simulink model "ASM_Traffic_V2X_Complete_Model_2"  (R2019a)
settings: Solver=ode1  StartTime=SIM.tstart.v  StopTime=Inf  FixedStep=SIM.StepSize.v  RelTol=1e-3
PostLoadFcn:
  | if any(exist('dsrtsu_mdlpostloadfcn', 'file') ~= 0), dsrtsu_mdlpostloadfcn('Execute', bdroot); end
  | try, asm_mdl_postloadfcn(bdroot, 'UpdateModel', 2200); catch, disp(lasterr); end,
undefined symbols (not defined in the file): _SensorPnts_1, _SensorPnts_13, _SensorPnts_17, _SensorPnts_21, _SensorPnts_25, _SensorPnts_29, _SensorPnts_33, _SensorPnts_37, _SensorPnts_41, _SensorPnts_45, _SensorPnts_49, _SensorPnts_5, _SensorPnts_53, _SensorPnts_57, _SensorPnts_9, _to_, CPT, G5A, ITS, MDL, rad, s_to_rpm, SIM
libraries: simulink x169, ASM_VehicleDynamics_lib x126, ASM_Traffic_lib x83, ASM_Utils_lib x49, mdbs x45, ASM_Environment_lib x17, dspindex x12, dsaV2xLibraryAux x10, dsmpblib x6, dsaV2xAsn1Library x4, dsaV2xLibrary x4, ASM_BrakeHydraulics_lib x4
(part 9 of 36)

== system ASM_Traffic_V2X_Complete_Model_2/MDLUserInterface/MotionDeskInterface/ASM_VehicleLights ==
  Environment : Inport
  VehDyn : Inport  Port=2
  Bus Selector : BusSelector  OutputSignals=Maneuver.UserSignals_Customized.ASM_Vehicle_TurnLights[]
  Bus Selector1 : BusSelector  OutputSignals=SW_ManualControl_Lights[1Maneuver|2Manual],SW_BrakeLight[0Off|1On],SW_TurnLights[0Off|1Left|2Right|3Both]
  Bus Selector3 : BusSelector  OutputSignals=Brake.BrakeDisc.Pressure.p_FL_Brake[bar],Brake.BrakeDisc.Pressure.p_FR_Brake[bar],Brake.BrakeDisc.Pressure.p_RL_Brake[bar],Brake.BrakeDisc.Pressure.p_RR_Brake[bar]
  Cmp_BrakePres : simulink/Logic and Bit Operations/Compare To Constant  relop=>  const=3  OutDataTypeStr=boolean
  Compare_Hazard : simulink/Logic and Bit Operations/Compare To Constant  relop===  const=3  OutDataTypeStr=boolean
  Compare_Turnlight_L : simulink/Logic and Bit Operations/Compare To Constant  relop===  const=1.0  OutDataTypeStr=boolean
  Compare_Turnlight_R : simulink/Logic and Bit Operations/Compare To Constant  relop===  const=2  OutDataTypeStr=boolean
  Data Type Conversion1 : DataTypeConversion  OutDataTypeStr=boolean
  Data Type Conversion2 : DataTypeConversion  OutDataTypeStr=uint32
  Data Type Conversion3 : DataTypeConversion  OutDataTypeStr=uint32
  Data Type Conversion4 : DataTypeConversion  OutDataTypeStr=uint32
  Gain : Gain  Gain=1/4
  Logical Operator : Logic  Operator=OR  AllPortsSameDT=off  OutDataTypeStr=boolean
  Logical Operator1 : Logic  Operator=OR  AllPortsSameDT=off  OutDataTypeStr=boolean
  Multiport Switch : MultiPortSwitch  Inputs=2
  Multiport Switch4 : MultiPortSwitch  Inputs=2
  Mux : Mux  Inputs=3
  Mux1 : Mux
  Sum of Elements : Sum  Inputs=+
  ASM_Vehicle_Lights[] : Outport
  wires:
  Mux/1 -> ASM_Vehicle_Lights[]/1
  Environment/1 -> Bus Selector/1
  Bus Selector/1 -> Data Type Conversion4/1  "<ASM_Vehicle_TurnLights[]>"
  Bus Selector1/1 -> Data Type Conversion3/1  "<SW_ManualControl_Lights[1Maneuver|2Manual]>"
  Bus Selector1/2 -> Data Type Conversion1/1  "<SW_BrakeLight[0Off|1On]>"
  Multiport Switch/1 -> Mux/1
  Compare_Turnlight_L/1 -> Logical Operator/1
  Compare_Turnlight_R/1 -> Logical Operator1/1
  Compare_Hazard/1 -> Logical Operator1/2, Logical Operator/2
  Logical Operator/1 -> Mux/2
  Logical Operator1/1 -> Mux/3
  Multiport Switch4/1 -> Compare_Turnlight_L/1, Compare_Turnlight_R/1, Compare_Hazard/1
  Bus Selector1/3 -> Data Type Conversion2/1  "<SW_TurnLights[0Off|1Left|2Right|3Both]>"
  [TAG_SW_ASMVehicleLights_Signals] -> Bus Selector1/1
  Data Type Conversion3/1 -> Multiport Switch/1, Multiport Switch4/1
  Data Type Conversion1/1 -> Multiport Switch/3
  Data Type Conversion2/1 -> Multiport Switch4/3
  Data Type Conversion4/1 -> Multiport Switch4/2
  VehDyn/1 -> Bus Selector3/1
  Cmp_BrakePres/1 -> Multiport Switch/2
  Bus Selector3/2 -> Mux1/2  "<p_FR_Brake[bar]>"
  Bus Selector3/4 -> Mux1/4  "<p_RR_Brake[bar]>"
  Bus Selector3/1 -> Mux1/1  "<p_FL_Brake[bar]>"
  Bus Selector3/3 -> Mux1/3  "<p_RL_Brake[bar]>"
  Sum of Elements/1 -> Gain/1
  Mux1/1 -> Sum of Elements/1
  Gain/1 -> Cmp_BrakePres/1

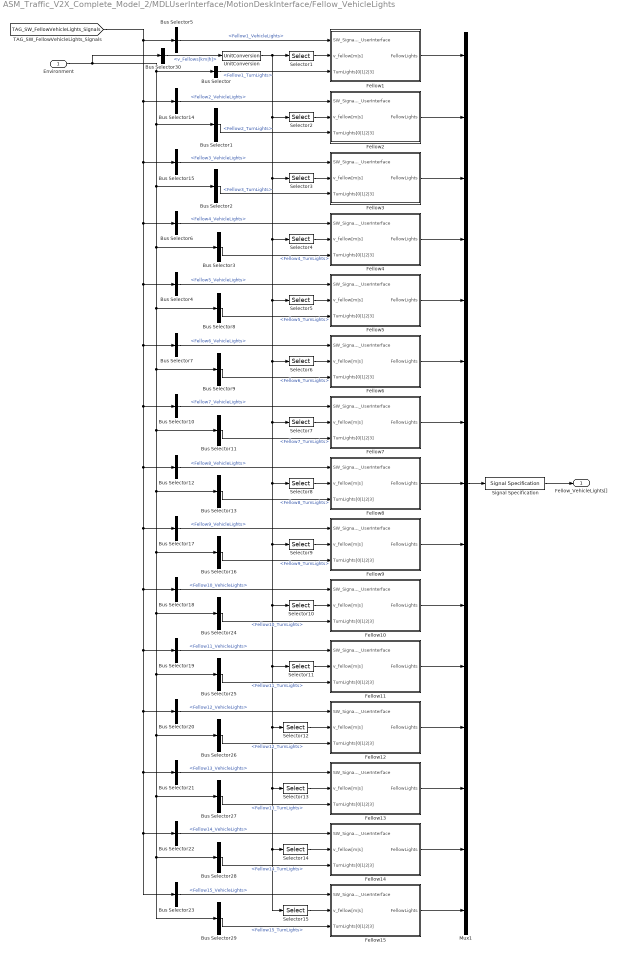
== system ASM_Traffic_V2X_Complete_Model_2/MDLUserInterface/MotionDeskInterface/Fellow_VehicleLights ==
  Environment : Inport
  Bus Selector : BusSelector  OutputSignals=Traffic.FellowMovement.UserSignals_Customized.Fellow1_TurnLights
  Bus Selector1 : BusSelector  OutputSignals=Traffic.FellowMovement.UserSignals_Customized.Fellow2_TurnLights
  Bus Selector10 : BusSelector  OutputSignals=Fellow7_VehicleLights
  Bus Selector11 : BusSelector  OutputSignals=Traffic.FellowMovement.UserSignals_Customized.Fellow7_TurnLights
  Bus Selector12 : BusSelector  OutputSignals=Fellow8_VehicleLights
  Bus Selector13 : BusSelector  OutputSignals=Traffic.FellowMovement.UserSignals_Customized.Fellow8_TurnLights
  Bus Selector14 : BusSelector  OutputSignals=Fellow2_VehicleLights
  Bus Selector15 : BusSelector  OutputSignals=Fellow3_VehicleLights
  Bus Selector16 : BusSelector  OutputSignals=Traffic.FellowMovement.UserSignals_Customized.Fellow9_TurnLights
  Bus Selector17 : BusSelector  OutputSignals=Fellow9_VehicleLights
  Bus Selector18 : BusSelector  OutputSignals=Fellow10_VehicleLights
  Bus Selector19 : BusSelector  OutputSignals=Fellow11_VehicleLights
  Bus Selector2 : BusSelector  OutputSignals=Traffic.FellowMovement.UserSignals_Customized.Fellow3_TurnLights
  Bus Selector20 : BusSelector  OutputSignals=Fellow12_VehicleLights
  Bus Selector21 : BusSelector  OutputSignals=Fellow13_VehicleLights
  Bus Selector22 : BusSelector  OutputSignals=Fellow14_VehicleLights
  Bus Selector23 : BusSelector  OutputSignals=Fellow15_VehicleLights
  Bus Selector24 : BusSelector  OutputSignals=Traffic.FellowMovement.UserSignals_Customized.Fellow10_TurnLights
  Bus Selector25 : BusSelector  OutputSignals=Traffic.FellowMovement.UserSignals_Customized.Fellow11_TurnLights
  Bus Selector26 : BusSelector  OutputSignals=Traffic.FellowMovement.UserSignals_Customized.Fellow12_TurnLights
  Bus Selector27 : BusSelector  OutputSignals=Traffic.FellowMovement.UserSignals_Customized.Fellow13_TurnLights
  Bus Selector28 : BusSelector  OutputSignals=Traffic.FellowMovement.UserSignals_Customized.Fellow14_TurnLights
  Bus Selector29 : BusSelector  OutputSignals=Traffic.FellowMovement.UserSignals_Customized.Fellow15_TurnLights
  Bus Selector3 : BusSelector  OutputSignals=Traffic.FellowMovement.UserSignals_Customized.Fellow4_TurnLights
  Bus Selector30 : BusSelector  OutputSignals=Traffic.FellowMovement.FellowMovement.v_Fellows[km|h]
  Bus Selector4 : BusSelector  OutputSignals=Fellow5_VehicleLights
  Bus Selector5 : BusSelector  OutputSignals=Fellow1_VehicleLights
  Bus Selector6 : BusSelector  OutputSignals=Fellow4_VehicleLights
  Bus Selector7 : BusSelector  OutputSignals=Fellow6_VehicleLights
  Bus Selector8 : BusSelector  OutputSignals=Traffic.FellowMovement.UserSignals_Customized.Fellow5_TurnLights
  Bus Selector9 : BusSelector  OutputSignals=Traffic.FellowMovement.UserSignals_Customized.Fellow6_TurnLights
  Fellow1 : Subsystem
  Fellow10 : Subsystem
  Fellow11 : Subsystem
  Fellow12 : Subsystem
  Fellow13 : Subsystem
  Fellow14 : Subsystem
  Fellow15 : Subsystem
  Fellow2 : Subsystem
  Fellow3 : Subsystem
  Fellow4 : Subsystem
  Fellow5 : Subsystem
  Fellow6 : Subsystem
  Fellow7 : Subsystem
  Fellow8 : Subsystem
  Fellow9 : Subsystem
  Mux1 : Mux  Inputs=15
  Selector1 : Selector  InputPortWidth=MDL.Traffic.MaxNumFellows.v  IndexOptions=Index vector (dialog)  Indices=1  OutputSizes=1
  Selector10 : Selector  InputPortWidth=MDL.Traffic.MaxNumFellows.v  IndexOptions=Index vector (dialog)  Indices=10  OutputSizes=1
  Selector11 : Selector  InputPortWidth=MDL.Traffic.MaxNumFellows.v  IndexOptions=Index vector (dialog)  Indices=11  OutputSizes=1
  Selector12 : Selector  InputPortWidth=MDL.Traffic.MaxNumFellows.v  IndexOptions=Index vector (dialog)  Indices=12  OutputSizes=1
  Selector13 : Selector  InputPortWidth=MDL.Traffic.MaxNumFellows.v  IndexOptions=Index vector (dialog)  Indices=13  OutputSizes=1
  Selector14 : Selector  InputPortWidth=MDL.Traffic.MaxNumFellows.v  IndexOptions=Index vector (dialog)  Indices=14  OutputSizes=1
  Selector15 : Selector  InputPortWidth=MDL.Traffic.MaxNumFellows.v  IndexOptions=Index vector (dialog)  Indices=15  OutputSizes=1
  Selector2 : Selector  InputPortWidth=MDL.Traffic.MaxNumFellows.v  IndexOptions=Index vector (dialog)  Indices=2  OutputSizes=1
  Selector3 : Selector  InputPortWidth=MDL.Traffic.MaxNumFellows.v  IndexOptions=Index vector (dialog)  Indices=3  OutputSizes=1
  Selector4 : Selector  InputPortWidth=MDL.Traffic.MaxNumFellows.v  IndexOptions=Index vector (dialog)  Indices=4  OutputSizes=1
  Selector5 : Selector  InputPortWidth=MDL.Traffic.MaxNumFellows.v  IndexOptions=Index vector (dialog)  Indices=5  OutputSizes=1
  Selector6 : Selector  InputPortWidth=MDL.Traffic.MaxNumFellows.v  IndexOptions=Index vector (dialog)  Indices=6  OutputSizes=1
  Selector7 : Selector  InputPortWidth=MDL.Traffic.MaxNumFellows.v  IndexOptions=Index vector (dialog)  Indices=7  OutputSizes=1
  Selector8 : Selector  InputPortWidth=MDL.Traffic.MaxNumFellows.v  IndexOptions=Index vector (dialog)  Indices=8  OutputSizes=1
  Selector9 : Selector  InputPortWidth=MDL.Traffic.MaxNumFellows.v  IndexOptions=Index vector (dialog)  Indices=9  OutputSizes=1
  Signal Specification : SignalSpecification  SampleTime=SIM.StepSize.v
  UnitConversion : ASM_Utils_lib/UnitConversion/UnitConversion  Selection=km/h_to_m/s
  Fellow_VehicleLights[] : Outport
  wires:
  UnitConversion/1 -> Selector1/1, Selector2/1, Selector3/1, Selector4/1, Selector5/1, Selector6/1, Selector7/1, Selector8/1, Selector9/1, Selector10/1, Selector11/1, Selector12/1, Selector13/1, Selector14/1, Selector15/1
  Bus Selector29/1 -> Fellow15/3(TurnLights[0|1|2|3])  "<Fellow15_TurnLights>"
  Bus Selector28/1 -> Fellow14/3(TurnLights[0|1|2|3])  "<Fellow14_TurnLights>"
  Bus Selector22/1 -> Fellow14/1(SW_Signals_UserInterface)  "<Fellow14_VehicleLights>"
  Bus Selector27/1 -> Fellow13/3(TurnLights[0|1|2|3])  "<Fellow13_TurnLights>"
  Bus Selector21/1 -> Fellow13/1(SW_Signals_UserInterface)  "<Fellow13_VehicleLights>"
  Bus Selector26/1 -> Fellow12/3(TurnLights[0|1|2|3])  "<Fellow12_TurnLights>"
  Bus Selector25/1 -> Fellow11/3(TurnLights[0|1|2|3])  "<Fellow11_TurnLights>"
  Bus Selector24/1 -> Fellow10/3(TurnLights[0|1|2|3])  "<Fellow10_TurnLights>"
  Bus Selector16/1 -> Fellow9/3(TurnLights[0|1|2|3])  "<Fellow9_TurnLights>"
  Bus Selector13/1 -> Fellow8/3(TurnLights[0|1|2|3])  "<Fellow8_TurnLights>"
  Bus Selector12/1 -> Fellow8/1(SW_Signals_UserInterface)  "<Fellow8_VehicleLights>"
  Bus Selector11/1 -> Fellow7/3(TurnLights[0|1|2|3])  "<Fellow7_TurnLights>"
  Bus Selector9/1 -> Fellow6/3(TurnLights[0|1|2|3])  "<Fellow6_TurnLights>"
  Bus Selector7/1 -> Fellow6/1(SW_Signals_UserInterface)  "<Fellow6_VehicleLights>"
  Bus Selector8/1 -> Fellow5/3(TurnLights[0|1|2|3])  "<Fellow5_TurnLights>"
  Bus Selector3/1 -> Fellow4/3(TurnLights[0|1|2|3])  "<Fellow4_TurnLights>"
  Bus Selector23/1 -> Fellow15/1(SW_Signals_UserInterface)  "<Fellow15_VehicleLights>"
  Bus Selector20/1 -> Fellow12/1(SW_Signals_UserInterface)  "<Fellow12_VehicleLights>"
  Bus Selector19/1 -> Fellow11/1(SW_Signals_UserInterface)  "<Fellow11_VehicleLights>"
  Bus Selector18/1 -> Fellow10/1(SW_Signals_UserInterface)  "<Fellow10_VehicleLights>"
  Fellow15/1(FellowLights) -> Mux1/15
  Fellow14/1(FellowLights) -> Mux1/14
  Fellow13/1(FellowLights) -> Mux1/13
  Fellow12/1(FellowLights) -> Mux1/12
  Fellow11/1(FellowLights) -> Mux1/11
  Fellow10/1(FellowLights) -> Mux1/10
  Bus Selector17/1 -> Fellow9/1(SW_Signals_UserInterface)  "<Fellow9_VehicleLights>"
  Bus Selector10/1 -> Fellow7/1(SW_Signals_UserInterface)  "<Fellow7_VehicleLights>"
  Bus Selector4/1 -> Fellow5/1(SW_Signals_UserInterface)  "<Fellow5_VehicleLights>"
  Bus Selector6/1 -> Fellow4/1(SW_Signals_UserInterface)  "<Fellow4_VehicleLights>"
  Bus Selector15/1 -> Fellow3/1(SW_Signals_UserInterface)  "<Fellow3_VehicleLights>"
  Bus Selector14/1 -> Fellow2/1(SW_Signals_UserInterface)  "<Fellow2_VehicleLights>"
  Bus Selector5/1 -> Fellow1/1(SW_Signals_UserInterface)  "<Fellow1_VehicleLights>"
  [TAG_SW_FellowVehicleLights_Signals] -> Bus Selector5/1, Bus Selector15/1, Bus Selector6/1, Bus Selector4/1, Bus Selector7/1, Bus Selector10/1, Bus Selector12/1, Bus Selector17/1, Bus Selector18/1, Bus Selector19/1, Bus Selector20/1, Bus Selector21/1, Bus Selector22/1, Bus Selector23/1, Bus Selector14/1
  Fellow9/1(FellowLights) -> Mux1/9
  Fellow8/1(FellowLights) -> Mux1/8
  Fellow7/1(FellowLights) -> Mux1/7
  Fellow6/1(FellowLights) -> Mux1/6
  Fellow5/1(FellowLights) -> Mux1/5
  Fellow4/1(FellowLights) -> Mux1/4
  Fellow3/1(FellowLights) -> Mux1/3
  Fellow2/1(FellowLights) -> Mux1/2
  Fellow1/1(FellowLights) -> Mux1/1
  Bus Selector2/1 -> Fellow3/3(TurnLights[0|1|2|3])  "<Fellow3_TurnLights>"
  Bus Selector1/1 -> Fellow2/3(TurnLights[0|1|2|3])  "<Fellow2_TurnLights>"
  Bus Selector/1 -> Fellow1/3(TurnLights[0|1|2|3])  "<Fellow1_TurnLights>"
  Environment/1 -> Bus Selector30/1, Bus Selector3/1, Bus Selector8/1, Bus Selector9/1, Bus Selector11/1, Bus Selector13/1, Bus Selector16/1, Bus Selector24/1, Bus Selector25/1, Bus Selector26/1, Bus Selector27/1, Bus Selector28/1, Bus Selector29/1, Bus Selector2/1, Bus Selector1/1, Bus Selector/1
  Mux1/1 -> Signal Specification/1
  Signal Specification/1 -> Fellow_VehicleLights[]/1
  Bus Selector30/1 -> UnitConversion/1  "<v_Fellows[km|h]>"
  Selector1/1 -> Fellow1/2(v_fellow[m|s])
  Selector2/1 -> Fellow2/2(v_fellow[m|s])
  Selector3/1 -> Fellow3/2(v_fellow[m|s])
  Selector4/1 -> Fellow4/2(v_fellow[m|s])
  Selector5/1 -> Fellow5/2(v_fellow[m|s])
  Selector6/1 -> Fellow6/2(v_fellow[m|s])
  Selector7/1 -> Fellow7/2(v_fellow[m|s])
  Selector8/1 -> Fellow8/2(v_fellow[m|s])
  Selector9/1 -> Fellow9/2(v_fellow[m|s])
  Selector10/1 -> Fellow10/2(v_fellow[m|s])
  Selector11/1 -> Fellow11/2(v_fellow[m|s])
  Selector12/1 -> Fellow12/2(v_fellow[m|s])
  Selector13/1 -> Fellow13/2(v_fellow[m|s])
  Selector14/1 -> Fellow14/2(v_fellow[m|s])
  Selector15/1 -> Fellow15/2(v_fellow[m|s])

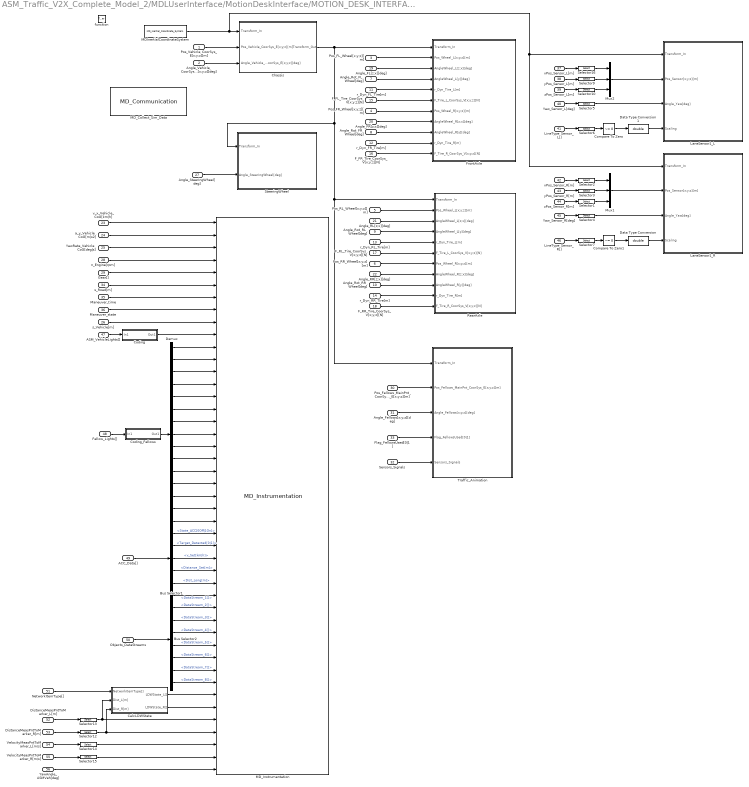
== system ASM_Traffic_V2X_Complete_Model_2/MDLUserInterface/MotionDeskInterface/MOTION_DESK_INTERFACE ==
  Pos_Vehicle_CoorSys_E[x;y;z][m] : Inport
  Angle_Vehicle_CoorSys_E[x;y;z][deg] : Inport  Port=2
  Pos_FL_Wheel[x;y;z][m] : Inport  Port=3
  Pos_FR_Wheel[x;y;z][m] : Inport  Port=4
  Pos_RL_Wheel[x;y;z][m] : Inport  Port=5
  Pos_RR_Wheel[x;y;z][m] : Inport  Port=6
  Angle_Rot_FL_Wheel[deg] : Inport  Port=7
  Angle_Rot_FR_Wheel[deg] : Inport  Port=8
  Angle_Rot_RL_Wheel[deg] : Inport  Port=9
  Angle_Rot_RR_Wheel[deg] : Inport  Port=10
  r_Dyn_FL_Tire[m] : Inport  Port=11
  r_Dyn_FR_Tire[m] : Inport  Port=12
  r_Dyn_RL_Tire[m] : Inport  Port=13
  r_Dyn_RR_Tire[m] : Inport  Port=14
  F_FL_Tire_CoorSys_V[x;y;z][N] : Inport  Port=15
  F_FR_Tire_CoorSys_V[x;y;z][N] : Inport  Port=16
  F_RL_Tire_CoorSys_V[x;y;z][N] : Inport  Port=17
  F_RR_Tire_CoorSys_V[x;y;z][N] : Inport  Port=18
  Angle_FL[z;x][deg] : Inport  Port=19
  Angle_FR[z;x][deg] : Inport  Port=20
  Angle_RL[z;x][deg] : Inport  Port=21
  Angle_RR[z;x][deg] : Inport  Port=22
  v_x_Vehicle_CoG[km|h] : Inport  Port=23
  a_y_Vehicle_CoG[m|s2] : Inport  Port=24
  YawRate_Vehicle_CoG[deg|s] : Inport  Port=25
  s_Vehicle[m] : Inport  Port=26
  Angle_SteeringWheel[deg] : Inport  Port=27
  n_Engine[rpm] : Inport  Port=28
  Gear[] : Inport  Port=29
  Pos_Fellows_MainPnt_CoorSys_E[x;y;z][m] : Inport  Port=30
  Angle_Fellows[x;y;z][deg] : Inport  Port=31
  Sensors_Signals : Inport  Port=32
  Flag_FellowsUsed[0|1] : Inport  Port=33
  s_Road[m] : Inport  Port=34
  Maneuver_time : Inport  Port=35
  Maneuver_state : Inport  Port=36
  xPos_Sensor_L[m] : Inport  Port=37
  yPos_Sensor_L[m] : Inport  Port=38
  zPos_Sensor_L[m] : Inport  Port=39
  Yaw_Sensor_L[deg] : Inport  Port=40
  LineType_Sensor_L[] : Inport  Port=41
  xPos_Sensor_R[m] : Inport  Port=42
  yPos_Sensor_R[m] : Inport  Port=43
  zPos_Sensor_R[m] : Inport  Port=44
  Yaw_Sensor_R[deg] : Inport  Port=45
  LineType_Sensor_R[] : Inport  Port=46
  ASM_VehicleLights[] : Inport  Port=47
  Fellow_Lights[] : Inport  Port=48
  ACC_Data[] : Inport  Port=49
  Objects_DataStreams : Inport  Port=50
  NetworkItemType[] : Inport  Port=51
  DistanceMeasPntToMarker_L[m] : Inport  Port=52
  DistanceMeasPntToMarker_R[m] : Inport  Port=53
  VelocityMeasPntToMarker_L[m/s] : Inport  Port=54
  VelocityMeasPntToMarker_R[m/s] : Inport  Port=55
  YawAngle_ASMVeh[deg] : Inport  Port=56
  function : TriggerPort  TriggerType=function-call  VariantControl=Variant
  Bus Selector1 : BusSelector  OutputSignals=Controller_ACC.State_ACC[0Off|1On],Target_Selection_ACC.Target_Detected[0|1],Controller_ACC.v_Set[km|h],Controller_ACC.Distance_Set[m],Target_Selection_ACC.Dist_Long[m]
  Bus Selector2 : BusSelector  OutputSignals=DataStream_1[].DataStream_1[],DataStream_2[].DataStream_2[],DataStream_3[].DataStream_3[],DataStream_4[].DataStream_4[],DataStream_5[].DataStream_5[],DataStream_6[].DataStream_6[],DataStream_7[].DataStream_7[],DataStream_8[].DataStream_8[]
  CalcLDWState : Subsystem
  Chassis : Subsystem
  Coding : Subsystem
  Coding_Fellows : Subsystem
  Compare To Zero : simulink/Logic and Bit Operations/Compare To Zero  relop=~=  OutDataTypeStr=uint8
  Compare To Zero1 : simulink/Logic and Bit Operations/Compare To Zero  relop=~=  OutDataTypeStr=uint8
  Data Type Conversion : DataTypeConversion  OutDataTypeStr=double
  Data Type Conversion1 : DataTypeConversion  OutDataTypeStr=double
  Demux : Demux  Outputs=15
  FrontAxle : Subsystem
  LaneSensor1_L : Subsystem
  LaneSensor1_R : Subsystem
  MDInertialCoordinateSystem : mdbs/MD_Inertial_Coordinate_System
      settings: SourceProductName=dSPACE MotionDesk Blockset
  MD_Collect_Sim_Data : mdbs/MD_Communication  bBlkRecSyncBld=0
      settings: SourceProductName=dSPACE MotionDesk Blockset
  MD_Instrumentation : mdbs/MD_Instrumentation  strNumDataStream=45  strToggleVal=0
      settings: SourceProductName=dSPACE MotionDesk Blockset
  Mux1 : Mux  Inputs=3
  Mux2 : Mux  Inputs=3
  RearAxle : Subsystem
  Selector{1..7,9..10,13..14,16} (12 alike) : Selector  IndexOptions=Index vector (dialog)  Indices=[1]  OutputSizes=1
  Selector12 : Selector  IndexOptions=Index vector (dialog)  Indices=[2]  OutputSizes=1
  Selector15 : Selector  IndexOptions=Index vector (dialog)  Indices=[2]  OutputSizes=1
  SteeringWheel : Subsystem
  Traffic_Animation : Subsystem
  wires:
  NetworkItemType[]/1 -> CalcLDWState/1(NetworkItemType[])
  CalcLDWState/2(LDWState_R[]) -> MD_Instrumentation/40
  CalcLDWState/1(LDWState_L[]) -> MD_Instrumentation/39
  YawAngle_ASMVeh[deg]/1 -> MD_Instrumentation/45
  Selector14/1 -> MD_Instrumentation/43
  Selector15/1 -> MD_Instrumentation/44
  Selector12/1 -> CalcLDWState/3(Dist_R[m]), MD_Instrumentation/42
  Selector13/1 -> MD_Instrumentation/41, CalcLDWState/2(Dist_L[m])
  VelocityMeasPntToMarker_R[m/s]/1 -> Selector15/1
  VelocityMeasPntToMarker_L[m/s]/1 -> Selector14/1
  DistanceMeasPntToMarker_R[m]/1 -> Selector12/1
  DistanceMeasPntToMarker_L[m]/1 -> Selector13/1
  Bus Selector2/8 -> MD_Instrumentation/38  "<DataStream_8[]>"
  Bus Selector2/6 -> MD_Instrumentation/36  "<DataStream_6[]>"
  Bus Selector2/7 -> MD_Instrumentation/37  "<DataStream_7[]>"
  Bus Selector2/3 -> MD_Instrumentation/33  "<DataStream_3[]>"
  Bus Selector2/1 -> MD_Instrumentation/31  "<DataStream_1[]>"
  Bus Selector2/2 -> MD_Instrumentation/32  "<DataStream_2[]>"
  Bus Selector2/4 -> MD_Instrumentation/34  "<DataStream_4[]>"
  Bus Selector2/5 -> MD_Instrumentation/35  "<DataStream_5[]>"
  Objects_DataStreams/1 -> Bus Selector2/1
  Bus Selector1/5 -> MD_Instrumentation/30  "<Dist_Long[m]>"
  Bus Selector1/4 -> MD_Instrumentation/29  "<Distance_Set[m]>"
  Bus Selector1/3 -> MD_Instrumentation/28  "<v_Set[km|h]>"
  Bus Selector1/2 -> MD_Instrumentation/27  "<Target_Detected[0|1]>"
  Bus Selector1/1 -> MD_Instrumentation/26  "<State_ACC[0Off|1On]>"
  ACC_Data[]/1 -> Bus Selector1/1
  s_Vehicle[m]/1 -> MD_Instrumentation/9
  Maneuver_state/1 -> MD_Instrumentation/8
  Maneuver_time/1 -> MD_Instrumentation/7
  s_Road[m]/1 -> MD_Instrumentation/6
  Gear[]/1 -> MD_Instrumentation/5
  n_Engine[rpm]/1 -> MD_Instrumentation/4
  YawRate_Vehicle_CoG[deg|s]/1 -> MD_Instrumentation/3
  a_y_Vehicle_CoG[m|s2]/1 -> MD_Instrumentation/2
  v_x_Vehicle_CoG[km|h]/1 -> MD_Instrumentation/1
  Angle_RL[z;x][deg]/1 -> RearAxle/3(AngleWheel_L[z;x][deg])
  Angle_FL[z;x][deg]/1 -> FrontAxle/3(AngleWheel_L[z;x][deg])
  Chassis/1(Transform_Out) -> Traffic_Animation/1(Transform_In), RearAxle/1(Transform_In), SteeringWheel/1(Transform_In), FrontAxle/1(Transform_In)
  MDInertialCoordinateSystem/1 -> Chassis/1(Transform_In), LaneSensor1_L/1(Transform_In), LaneSensor1_R/1(Transform_In)
  Pos_FR_Wheel[x;y;z][m]/1 -> FrontAxle/7(Pos_Wheel_R[x;y;z][m])
  Angle_FR[z;x][deg]/1 -> FrontAxle/8(AngleWheel_R[z;x][deg])
  Angle_Rot_FR_Wheel[deg]/1 -> FrontAxle/9(AngleWheel_R[y][deg])
  r_Dyn_FR_Tire[m]/1 -> FrontAxle/10(r_Dyn_Tire_R[m])
  F_FR_Tire_CoorSys_V[x;y;z][N]/1 -> FrontAxle/11(F_Tire_R_CoorSys_V[x;y;z][N])
  Pos_FL_Wheel[x;y;z][m]/1 -> FrontAxle/2(Pos_Wheel_L[x;y;z][m])
  Angle_Rot_FL_Wheel[deg]/1 -> FrontAxle/4(AngleWheel_L[y][deg])
  r_Dyn_FL_Tire[m]/1 -> FrontAxle/5(r_Dyn_Tire_L[m])
  F_FL_Tire_CoorSys_V[x;y;z][N]/1 -> FrontAxle/6(F_Tire_L_CoorSys_V[x;y;z][N])
  Pos_RL_Wheel[x;y;z][m]/1 -> RearAxle/2(Pos_Wheel_L[x;y;z][m])
  Angle_Rot_RL_Wheel[deg]/1 -> RearAxle/4(AngleWheel_L[y][deg])
  r_Dyn_RL_Tire[m]/1 -> RearAxle/5(r_Dyn_Tire_L[m])
  F_RL_Tire_CoorSys_V[x;y;z][N]/1 -> RearAxle/6(F_Tire_L_CoorSys_V[x;y;z][N])
  F_RR_Tire_CoorSys_V[x;y;z][N]/1 -> RearAxle/11(F_Tire_R_CoorSys_V[x;y;z][N])
  r_Dyn_RR_Tire[m]/1 -> RearAxle/10(r_Dyn_Tire_R[m])
  Angle_Rot_RR_Wheel[deg]/1 -> RearAxle/9(AngleWheel_R[y][deg])
  Angle_RR[z;x][deg]/1 -> RearAxle/8(AngleWheel_R[z;x][deg])
  Pos_RR_Wheel[x;y;z][m]/1 -> RearAxle/7(Pos_Wheel_R[x;y;z][m])
  Pos_Vehicle_CoorSys_E[x;y;z][m]/1 -> Chassis/2(Pos_Vehicle_CoorSys_E[x;y;z][m])
  Angle_Vehicle_CoorSys_E[x;y;z][deg]/1 -> Chassis/3(Angle_Vehicle_CoorSys_E[x;y;z][deg])
  Angle_SteeringWheel[deg]/1 -> SteeringWheel/2(Angle_SteeringWheel[deg])
  Pos_Fellows_MainPnt_CoorSys_E[x;y;z][m]/1 -> Traffic_Animation/2(Pos_Fellows_MainPnt_CoorSys_E[x;y;z][m])
  Angle_Fellows[x;y;z][deg]/1 -> Traffic_Animation/3(Angle_Fellows[x;y;z][deg])
  Flag_FellowsUsed[0|1]/1 -> Traffic_Animation/4(Flag_FellowsUsed[0|1])
  Yaw_Sensor_L[deg]/1 -> Selector5/1
  Yaw_Sensor_R[deg]/1 -> Selector4/1
  Selector16/1 -> Mux2/1
  Selector9/1 -> Mux2/2
  Selector10/1 -> Mux2/3
  xPos_Sensor_L[m]/1 -> Selector16/1
  yPos_Sensor_L[m]/1 -> Selector9/1
  zPos_Sensor_L[m]/1 -> Selector10/1
  Mux2/1 -> LaneSensor1_L/2(Pos_Sensor[x;y;z][m])
  Selector2/1 -> Mux1/1
  Selector3/1 -> Mux1/2
  Selector1/1 -> Mux1/3
  Mux1/1 -> LaneSensor1_R/2(Pos_Sensor[x;y;z][m])
  xPos_Sensor_R[m]/1 -> Selector2/1
  yPos_Sensor_R[m]/1 -> Selector3/1
  zPos_Sensor_R[m]/1 -> Selector1/1
  Selector4/1 -> LaneSensor1_R/3(Angle_Yaw[deg])
  Selector5/1 -> LaneSensor1_L/3(Angle_Yaw[deg])
  LineType_Sensor_L[]/1 -> Selector6/1
  Compare To Zero/1 -> Data Type Conversion1/1
  Selector6/1 -> Compare To Zero/1
  Selector7/1 -> Compare To Zero1/1
  LineType_Sensor_R[]/1 -> Selector7/1
  Compare To Zero1/1 -> Data Type Conversion/1
  Data Type Conversion/1 -> LaneSensor1_R/4(Scaling)
  Data Type Conversion1/1 -> LaneSensor1_L/4(Scaling)
  ASM_VehicleLights[]/1 -> Coding/1(In1)
  Fellow_Lights[]/1 -> Coding_Fellows/1(In1)
  Coding_Fellows/1(Out1) -> Demux/1
  Coding/1(Out1) -> MD_Instrumentation/10
  Demux/1 -> MD_Instrumentation/11
  Demux/2 -> MD_Instrumentation/12
  Demux/3 -> MD_Instrumentation/13
  Demux/4 -> MD_Instrumentation/14
  Demux/5 -> MD_Instrumentation/15
  Demux/6 -> MD_Instrumentation/16
  Demux/7 -> MD_Instrumentation/17
  Demux/8 -> MD_Instrumentation/18
  Demux/9 -> MD_Instrumentation/19
  Demux/10 -> MD_Instrumentation/20
  Demux/11 -> MD_Instrumentation/21
  Demux/12 -> MD_Instrumentation/22
  Demux/13 -> MD_Instrumentation/23
  Demux/14 -> MD_Instrumentation/24
  Demux/15 -> MD_Instrumentation/25
  Sensors_Signals/1 -> Traffic_Animation/5(Sensors_Signals)

== system ASM_Traffic_V2X_Complete_Model_2/MDLUserInterface/MotionDeskInterface/OpenMotionDeskInterfaceModel ==

== system ASM_Traffic_V2X_Complete_Model_2/MDLUserInterface/SoftECU/MDL_DISP ==
  Bus Selector2 : BusSelector  OutputSignals=SoftECU_Engine,SoftECU_Brake,SoftECU_ACC,SoftECU_Transmission,SoftECU_StartButton
  SoftECU_ACC : Subsystem
  SoftECU_Body : Subsystem
  SoftECU_Brake : Subsystem
  SoftECU_Engine : Subsystem
  SoftECU_Transmission : Subsystem
  wires:
  [ASMBUS_SoftECU] -> Bus Selector2/1
  Bus Selector2/4 -> SoftECU_Transmission/1(ASMSignalBus)  "<SoftECU_Transmission>"
  Bus Selector2/1 -> SoftECU_Engine/1(ASMSignalBus)  "<SoftECU_Engine>"
  Bus Selector2/2 -> SoftECU_Brake/1(ASMSignalBus)  "<SoftECU_Brake>"
  Bus Selector2/3 -> SoftECU_ACC/1(ASMSignalBus_ACC)  "<SoftECU_ACC>"
  [ASMBUS_VehicleDynamics] -> SoftECU_ACC/2(ASMSignalBus_Vehicle)
  Bus Selector2/5 -> SoftECU_Body/1(In)  "<SoftECU_StartButton>"

== system ASM_Traffic_V2X_Complete_Model_2/MDLUserInterface/SoftECU/MDL_PAR ==
  Bus Creator : BusCreator  Inputs=9
  SoftECU_ESP_Switches : Subsystem
      mask Display: disp('SoftECU ESP Switches')
  SoftECU_StartButton_Switches : Subsystem
      mask Display: disp('SoftECU Start Button Switches')
  Sw_ACC_BrakeMode[1Comfort|2AEBOnly|3AEBOff] : Constant  Value=3
  Sw_ACC_Cancel[0Off|1On] : Constant  Value=0
  Sw_ACC_Control_Mode[1ManSched|2Manual] : Constant
  Sw_ACC_Off[0Off|1On] : Constant  Value=0
  Sw_ACC_On[0Off|1On] : Constant  Value=0
  Sw_ACC_Resume[0Off|1On] : Constant  Value=0
  Sw_ACC_Speed_Decrease[0Off|1On] : Constant  Value=0
  Sw_ACC_Speed_Increase[0Off|1On] : Constant  Value=0
  Sw_ACC_Speed_Set[0Off|1On] : Constant  Value=0
  tag scope: TAG_SoftECU_Switches_ACC=global
  wires:
  Sw_ACC_Control_Mode[1ManSched|2Manual]/1 -> Bus Creator/1  "Sw_ACC_Control_Mode[1ManSched|2Manual]"
  Sw_ACC_On[0Off|1On]/1 -> Bus Creator/2  "Sw_ACC_On[Off|1On]"
  Sw_ACC_Off[0Off|1On]/1 -> Bus Creator/3  "Sw_ACC_Off[0Off|1On]"
  Sw_ACC_Cancel[0Off|1On]/1 -> Bus Creator/4  "Sw_ACC_Cancel[0Off|1On]"
  Sw_ACC_Resume[0Off|1On]/1 -> Bus Creator/5  "Sw_ACC_Resume[0Off|1On]"
  Sw_ACC_Speed_Set[0Off|1On]/1 -> Bus Creator/6  "Sw_ACC_Speed_Set[0Off|1On]"
  Sw_ACC_Speed_Increase[0Off|1On]/1 -> Bus Creator/7  "Sw_ACC_Speed_Increase[0Off|1On]"
  Sw_ACC_Speed_Decrease[0Off|1On]/1 -> Bus Creator/8  "Sw_ACC_Speed_Decrease[0Off|1On]"
  Bus Creator/1 -> [TAG_SoftECU_Switches_ACC]  "Switches_ACC"
  Sw_ACC_BrakeMode[1Comfort|2AEBOnly|3AEBOff]/1 -> Bus Creator/9  "Sw_ACC_BrakeMode[1Comfort|2AEBOnly|3AEBOff]"

== system ASM_Traffic_V2X_Complete_Model_2/MDLUserInterface/SoftECU/MDL_TEST ==

== system ASM_Traffic_V2X_Complete_Model_2/MDLUserInterface/VehicleDynamics/MDL_DISP ==
  Accelerations : Subsystem
  Aerodynamics : Subsystem
  Brake : Subsystem
  Bus Selector2 : BusSelector  OutputSignals=VehicleMovement.Positions,VehicleMovement.Velocities,VehicleMovement.Accelerations,Wheel,Tire,Aerodynamics,Steering,Brake
  Overview : Subsystem
  Positions : Subsystem
  Steering : Subsystem
  Suspension : Subsystem
      mask Display: disp('Suspension')
  Tire : Subsystem
  Velocities : Subsystem
  WheelSpeeds : Subsystem
  wires:
  Bus Selector2/8 -> Brake/1(Brake)  "<Brake>"
  Bus Selector2/7 -> Steering/1(Steering)  "<Steering>"
  Bus Selector2/6 -> Aerodynamics/1(Aerodynamics)  "<Aerodynamics>"
  Bus Selector2/5 -> Tire/1(Tire)  "<Tire>"
  Bus Selector2/3 -> Accelerations/1(Accelerations), Overview/2(Accelerations)  "<Accelerations>"
  Bus Selector2/2 -> Velocities/1(Velocities), Overview/1(Velocities)  "<Velocities>"
  Bus Selector2/1 -> Positions/1(Positions)  "<Positions>"
  Bus Selector2/4 -> WheelSpeeds/1(WheelSpeeds)  "<Wheel>"
  [ASMBUS_VehicleDynamics] -> Bus Selector2/1

== system ASM_Traffic_V2X_Complete_Model_2/MDLUserInterface/VehicleDynamics/MDL_PAR ==
  BRAKE_HYDRAULICS_VARIANT_SWITCHES : ASM_BrakeHydraulics_lib/BrakeHydraulics/BRAKE_HYDRAULICS_VARIANT_SWITCHES  Tag=ASM_SUBCOMPONENT  SW_MasterBrakeCylinder_Mode=MDL.BrkHyd.SW_MasterBrakeCylinderType.v  ASMProperties=struct('Name','BRAKE_HYDRAULICS_VARIANT_SWITCHES','Version','4.0','Library','ASM_BrakeHydraulics_lib')  ASMInstanceName=MasterBrakeCylinder  ASMInstanceID=1
  BrakeHydraulics_DistributionPattern_Switch : Subsystem
      mask Display: disp('BrakeHydraulics_DistributionPattern_Switch')
  ROTATION_SWITCH : ASM_VehicleDynamics_lib/VehicleDynamics/Suspension/Common/ROTATION_SWITCH  Tag=ASM_SUBCOMPONENT  Sw_Rotation=MDL.VehicleDynamics.SW_Rotation  ASMProperties=struct('Name','ROTATION_SWITCH','Version','2.0','Library','ASM_VehicleDynamics_lib')  ASMInstanceName=rotation_switch  ASMInstanceID=1
  Suspension_Inits : Subsystem
      mask Display: disp('Suspension Inits')
  Tire_Switches : Subsystem
      mask Display: disp('Tire Switches')
  VEHICLE_DYNAMICS_VARIANT_SWITCHES : ASM_VehicleDynamics_lib/VehicleDynamics/VEHICLE_DYNAMICS_VARIANT_SWITCHES  Tag=ASM_SUBCOMPONENT  SW_Tire_Model=MDL.VehicleDynamics.SW_Tire_Model.v  ASMProperties=struct('Name','VEHICLE_DYNAMICS_VARIANT_SWITCHES','Version','1.0','Library','ASM_VehicleDynamics_lib')  ASMInstanceName=vehicle_dynamics_variant_switches  ASMInstanceID=1
  tag scope: TAG_SW_Rotation=global, TAG_Sw_MasterBrakeCylinder_Mode=global
  wires:
  BRAKE_HYDRAULICS_VARIANT_SWITCHES/1 -> [TAG_Sw_MasterBrakeCylinder_Mode]
  ROTATION_SWITCH/1 -> [TAG_SW_Rotation]

== system ASM_Traffic_V2X_Complete_Model_2/MDLUserInterface/VehicleDynamics/MDL_TEST ==

== system ASM_Traffic_V2X_Complete_Model_2/IO/I//O_Subsystem/Bus Configuration (1) - In/Simulated ECUs ==
  Input : Inport
  DrivekitCAN : Subsystem
  _Simulated ECUs_ : BusCreator  Inputs=1
  Simulated ECUs : Outport
  wires:
  _Simulated ECUs_/1 -> Simulated ECUs/1  "Simulated ECUs"
  DrivekitCAN/1(DrivekitCAN) -> _Simulated ECUs_/1  "DrivekitCAN"
  Input/1 -> DrivekitCAN/1(Input)

== system ASM_Traffic_V2X_Complete_Model_2/IO/I//O_Subsystem/Bus Configuration (1) - Out/Simulated ECUs ==
  Simulated ECUs : Inport
  DrivekitCAN : Subsystem
  _Simulated ECUs_ : BusSelector  OutputSignals=DrivekitCAN
  wires:
  Simulated ECUs/1 -> _Simulated ECUs_/1  "Simulated ECUs"
  _Simulated ECUs_/1 -> DrivekitCAN/1(DrivekitCAN)  "<DrivekitCAN>"

== system ASM_Traffic_V2X_Complete_Model_2/IO/I//O_Subsystem/EgoCar_Data/GPS ==
  In1 : Inport
  Bus Creator : BusCreator  Inputs=3
  Bus Selector : BusSelector  OutputSignals=Environment.Road.Pos_Vehicle_GPS[Long;Lat][deg].Latitude[deg],Environment.Road.Pos_Vehicle_GPS[Long;Lat][deg].Longitude[deg],VehicleDynamics.VehicleMovement.Positions.Vehicle.Angular.Angle_Vehicle_CoorSys_E[x;y;z][deg].Angle_Yaw_Vehicle_CoorSys_E[deg]
  Gain : Gain
  Gain1 : Gain
  Gain2 : Gain
  MATLAB Function : MATLAB Function  TreatAsAtomicUnit=on
  Out1 : Outport
  wires:
  Bus Creator/1 -> Out1/1
  MATLAB Function/1(y) -> Gain2/1
  Gain2/1 -> Bus Creator/3  "Heading Value"
  Bus Selector/3 -> MATLAB Function/1(u)  "<Angle_Yaw_Vehicle_CoorSys_E[deg]>"
  Gain1/1 -> Bus Creator/2  "Long Value"
  Bus Selector/2 -> Gain1/1  "<Longitude[deg]>"
  Bus Selector/1 -> Gain/1  "<Latitude[deg]>"
  Gain/1 -> Bus Creator/1  "Lat Value"
  In1/1 -> Bus Selector/1

== system ASM_Traffic_V2X_Complete_Model_2/IO/I//O_Subsystem/EgoCar_Data/Lane_Number ==
  In1 : Inport
  Bus Selector : BusSelector  OutputSignals=Environment.Driver.LateralController.signal2.laneNumber,Environment.Road.LaneSensor_Dynamic.Sensor_Output.CurrentLane
  Gain : Gain  Gain=1/100
  Gain2 : Gain
  Terminator : Terminator
  Out1 : Outport
  wires:
  In1/1 -> Bus Selector/1
  Bus Selector/1 -> Gain/1  "<laneNumber>"
  Gain2/1 -> Terminator/1  "laneNumber"
  Gain/1 -> Gain2/1
  Bus Selector/2 -> Out1/1  "<CurrentLane>"

== system ASM_Traffic_V2X_Complete_Model_2/IO/I//O_Subsystem/EgoCar_Data/Steering_Angle ==
  In1 : Inport
  Bus Selector : BusSelector  OutputSignals=Environment.Driver.OutputSignals.Angle_SteeringWheel[deg]
  Gain : Gain
  Out1 : Outport
  wires:
  In1/1 -> Bus Selector/1
  Gain/1 -> Out1/1  "SAS_Angle Value"
  Bus Selector/1 -> Gain/1  "<Angle_SteeringWheel[deg]>"

== system ASM_Traffic_V2X_Complete_Model_2/IO/I//O_Subsystem/EgoCar_Data/Wheel_Speed ==
  In1 : Inport
  Bus Creator : BusCreator  Inputs=4
  Bus Selector : BusSelector  OutputSignals=VehicleDynamics.Wheel.WheelSpeed.omega_RR_Wheel[rad|s],VehicleDynamics.Wheel.WheelSpeed.omega_RL_Wheel[rad|s],VehicleDynamics.Wheel.WheelSpeed.omega_FR_Wheel[rad|s],VehicleDynamics.Wheel.WheelSpeed.omega_FL_Wheel[rad|s]
  Gain{,1..3} (4 alike) : Gain
  km/h_conversion{,1..3} (4 alike) : Gain  Gain=0.36*3.6
  Out1 : Outport
  wires:
  Bus Creator/1 -> Out1/1
  Gain3/1 -> Bus Creator/4  "WHL_SPD_FL Value"
  km/h_conversion3/1 -> Gain3/1
  km/h_conversion2/1 -> Gain2/1
  Gain2/1 -> Bus Creator/3  "WHL_SPD_FR Value"
  km/h_conversion1/1 -> Gain1/1
  Gain1/1 -> Bus Creator/2  "WHL_SPD_RL Value"
  Gain/1 -> Bus Creator/1  "WHL_SPD_RR Value"
  km/h_conversion/1 -> Gain/1
  Bus Selector/1 -> km/h_conversion/1  "<omega_RR_Wheel[rad|s]>"
  Bus Selector/4 -> km/h_conversion3/1  "<omega_FL_Wheel[rad|s]>"
  Bus Selector/2 -> km/h_conversion1/1  "<omega_RL_Wheel[rad|s]>"
  In1/1 -> Bus Selector/1
  Bus Selector/3 -> km/h_conversion2/1  "<omega_FR_Wheel[rad|s]>"

== system ASM_Traffic_V2X_Complete_Model_2/IO/V2X_Subsystem/CAM-DENM_Message_Generation/DENM ==
  note: Alternative DENM Transmission as UDP over Erthernet to Control PC
  "GENDENMData " : Inport
  Alternative_UDP2ControlPC_Directly : Subsystem
  Create_DENM : Subsystem
  DENM_Encode : Subsystem
  DENM_FREQ : DiscretePulseGenerator  PulseType=Time based  Period=0.2  PulseWidth=50
  DENM_trigger_Conditions : Subsystem
  Terminator : Terminator
  UDP_Trigger : Subsystem
  denm_freq : Outport
  denm : Outport  Port=2
  wires:
  DENM_FREQ/1 -> DENM_Encode/Trigger, denm_freq/1
  DENM_Encode/1(OutputDENM) -> denm/1
  Create_DENM/1(DENM1) -> DENM_Encode/1(DENM)
  "GENDENMData "/1 -> UDP_Trigger/1(In1), DENM_trigger_Conditions/1(In1)
  UDP_Trigger/1(Out1) -> Terminator/1
  DENM_trigger_Conditions/1(Out1) -> Alternative_UDP2ControlPC_Directly/Trigger

== system ASM_Traffic_V2X_Complete_Model_2/IO/V2X_Subsystem/CAM-DENM_Message_Generation/Fellow_CAM_1 ==
  Input : Inport
  Bus Selector : BusSelector  OutputSignals=Longitude[deg],Latitude[deg],Speed,Heading,Fellow_ID,Enable
  CAM_Encode : Subsystem
  Clock : Clock
  Constant : Constant
  Create_CAM : Subsystem
  Data Type Conversion3 : DataTypeConversion
  F_Heading : Display
      settings: Decimation=6
  F_ID : Display
      settings: Decimation=6
  F_Lat : Display
      settings: Decimation=6
  F_Lon : Display
      settings: Decimation=6
  F_Speed : Display
      settings: Decimation=6
  Gain : Gain  Gain=1000
  Heading : Constant  Value=5
  ID : Constant  Value=10
  Latitude [deg] : Constant  Value=5
  Logical Operator : Logic  AllPortsSameDT=off  OutDataTypeStr=boolean
  Longitude [deg] : Constant  Value=5
  Speed [m/s] : Constant  Value=5
  Terminator{,1..5} (6 alike) : Terminator
  Data : Outport
  Bytes : Outport  Port=2
  Output_Enabler : Outport  Port=3
  wires:
  CAM_Encode/1(Data) -> Data/1
  Gain/1 -> Create_CAM/1(Time [s])
  Logical Operator/1 -> CAM_Encode/Trigger
  CAM_Encode/2(Bytes) -> Bytes/1
  Speed [m/s]/1 -> Terminator/1
  Latitude [deg]/1 -> Terminator2/1
  ID/1 -> Terminator4/1
  Heading/1 -> Terminator3/1
  Create_CAM/3("Output_Enabler ") -> Logical Operator/2
  Clock/1 -> Gain/1
  Constant/1 -> Data Type Conversion3/1
  Create_CAM/1(Send CAM) -> Logical Operator/1  "cam_trigger"
  Create_CAM/2(CAM) -> CAM_Encode/1(" CAM")
  Data Type Conversion3/1 -> Output_Enabler/1, Create_CAM/7(Enabler)
  Longitude [deg]/1 -> Terminator1/1
  Input/1 -> Bus Selector/1
  Bus Selector/1 -> F_Lon/1, Create_CAM/2(Latitude [deg])  "<Longitude[deg]>"
  Bus Selector/2 -> Create_CAM/3(Longitude [deg]), F_Lat/1  "<Latitude[deg]>"
  Bus Selector/3 -> F_Speed/1, Create_CAM/4(Speed [km/h])  "<Speed>"
  Bus Selector/4 -> F_Heading/1, Create_CAM/5(Direction)  "<Heading>"
  Bus Selector/5 -> F_ID/1, Create_CAM/6(Fellow_ID)  "<Fellow_ID>"
  Bus Selector/6 -> Terminator5/1  "<Enable>"

== system ASM_Traffic_V2X_Complete_Model_2/IO/V2X_Subsystem/CAM-DENM_Message_Generation/Fellow_CAM_2 ==
  Input : Inport
  Bus Selector : BusSelector  OutputSignals=Longitude[deg],Latitude[deg],Speed,Heading,Fellow_ID,Enable
  CAM_Encode : Subsystem
  Clock : Clock
  Constant : Constant
  Create_CAM : Subsystem
  Data Type Conversion3 : DataTypeConversion
  F_Heading : Display
      settings: Decimation=6
  F_ID : Display
      settings: Decimation=6
  F_Lat : Display
      settings: Decimation=6
  F_Lon : Display
      settings: Decimation=6
  F_Speed : Display
      settings: Decimation=6
  Gain : Gain  Gain=1000
  Heading : Constant  Value=5
  ID : Constant  Value=10
  Latitude [deg] : Constant  Value=5
  Logical Operator : Logic  AllPortsSameDT=off  OutDataTypeStr=boolean
  Longitude [deg] : Constant  Value=5
  Speed [m/s] : Constant  Value=5
  Terminator{,1..5} (6 alike) : Terminator
  Data : Outport
  Bytes : Outport  Port=2
  Output_Enabler : Outport  Port=3
  wires:
  CAM_Encode/1(Data) -> Data/1
  Gain/1 -> Create_CAM/1(Time [s])
  Logical Operator/1 -> CAM_Encode/Trigger
  CAM_Encode/2(Bytes) -> Bytes/1
  Speed [m/s]/1 -> Terminator/1
  Latitude [deg]/1 -> Terminator2/1
  ID/1 -> Terminator4/1
  Heading/1 -> Terminator3/1
  Create_CAM/3("Output_Enabler ") -> Logical Operator/2
  Clock/1 -> Gain/1
  Constant/1 -> Data Type Conversion3/1
  Create_CAM/1(Send CAM) -> Logical Operator/1  "cam_trigger"
  Create_CAM/2(CAM) -> CAM_Encode/1(" CAM")
  Data Type Conversion3/1 -> Output_Enabler/1, Create_CAM/7(Enabler)
  Longitude [deg]/1 -> Terminator1/1
  Input/1 -> Bus Selector/1
  Bus Selector/1 -> F_Lon/1, Create_CAM/2(Latitude [deg])  "<Longitude[deg]>"
  Bus Selector/2 -> Create_CAM/3(Longitude [deg]), F_Lat/1  "<Latitude[deg]>"
  Bus Selector/3 -> F_Speed/1, Create_CAM/4(Speed [km/h])  "<Speed>"
  Bus Selector/4 -> F_Heading/1, Create_CAM/5(Direction)  "<Heading>"
  Bus Selector/5 -> F_ID/1, Create_CAM/6(Fellow_ID)  "<Fellow_ID>"
  Bus Selector/6 -> Terminator5/1  "<Enable>"

== system ASM_Traffic_V2X_Complete_Model_2/IO/V2X_Subsystem/CAM-DENM_Message_Generation/Fellow_CAM_3 ==
  Input : Inport
  Bus Selector : BusSelector  OutputSignals=Latitude[deg],Longitude[deg],Speed,Heading,Fellow_ID,Enable
  CAM_Encode : Subsystem
  Clock : Clock
  Constant : Constant
  Create_CAM : Subsystem
  Data Type Conversion3 : DataTypeConversion
  Gain : Gain  Gain=1000
  Logical Operator : Logic  AllPortsSameDT=off  OutDataTypeStr=boolean
  Terminator5 : Terminator
  Data : Outport
  Bytes : Outport  Port=2
  Output_Enabler : Outport  Port=3
  wires:
  CAM_Encode/1(Data) -> Data/1
  Gain/1 -> Create_CAM/1(Time [s])
  Logical Operator/1 -> CAM_Encode/Trigger
  CAM_Encode/2(Bytes) -> Bytes/1
  Create_CAM/3("Output_Enabler ") -> Logical Operator/2
  Clock/1 -> Gain/1
  Constant/1 -> Data Type Conversion3/1
  Create_CAM/1(Send CAM) -> Logical Operator/1  "cam_trigger"
  Create_CAM/2(CAM) -> CAM_Encode/1(" CAM")
  Data Type Conversion3/1 -> Output_Enabler/1, Create_CAM/7(Enabler)
  Input/1 -> Bus Selector/1
  Bus Selector/2 -> Create_CAM/3(Longitude [deg])  "<Longitude[deg]>"
  Bus Selector/1 -> Create_CAM/2(Latitude [deg])  "<Latitude[deg]>"
  Bus Selector/3 -> Create_CAM/4(Speed [km/h])  "<Speed>"
  Bus Selector/4 -> Create_CAM/5(Direction)  "<Heading>"
  Bus Selector/5 -> Create_CAM/6(Fellow_ID)  "<Fellow_ID>"
  Bus Selector/6 -> Terminator5/1  "<Enable>"

== system ASM_Traffic_V2X_Complete_Model_2/IO/V2X_Subsystem/CAM-DENM_Message_Generation/Queue_CAM ==
  Fellow_1 : Inport
  Fellow_2 : Inport  Port=2
  Fellow_3 : Inport  Port=3
  Enable_CAM1 : Inport  Port=4
  Enable_CAM2 : Inport  Port=5
  Enable_CAM3 : Inport  Port=6
  Enable : EnablePort  StatesWhenEnabling=reset
  Add : Sum
  Constant9 : Constant
  Demux : Demux  Outputs=1
  MATLAB Function : MATLAB Function  TreatAsAtomicUnit=on
  MATLAB Function1 : MATLAB Function  TreatAsAtomicUnit=on
  Unit Delay : UnitDelay  SampleTime=-1
  OutputCAM : Outport
  wires:
  Fellow_1/1 -> MATLAB Function/1(cam1)
  Constant9/1 -> Add/1
  MATLAB Function1/1(z) -> MATLAB Function/7(z)
  Add/1 -> Unit Delay/1, MATLAB Function1/1(p)
  Unit Delay/1 -> Add/2
  MATLAB Function/1(outvectorcam) -> Demux/1
  Enable_CAM1/1 -> MATLAB Function/2(e1)
  Fellow_2/1 -> MATLAB Function/3(cam2)
  Fellow_3/1 -> MATLAB Function/5(cam3)
  Enable_CAM2/1 -> MATLAB Function/4(e2)
  Enable_CAM3/1 -> MATLAB Function/6(e3)
  Demux/1 -> OutputCAM/1

== system ASM_Traffic_V2X_Complete_Model_2/IO/V2X_Subsystem/CAM-DENM_Message_Generation/Queue_CAM_DENM ==
  cam : Inport
  denm : Inport  Port=2
  Enable_CAM : Inport  Port=3
  Enable_DENM : Inport  Port=4
  Trigger : TriggerPort  VariantControl=Variant  PortDimensions=1
  Add : Sum
  Constant9 : Constant
  Demux : Demux  Outputs=2
  MATLAB Function : MATLAB Function  TreatAsAtomicUnit=on
  MATLAB Function2 : MATLAB Function  TreatAsAtomicUnit=on
  Unit Delay : UnitDelay  SampleTime=-1
  Data : Outport
  Byte : Outport  Port=2
  wires:
  Enable_DENM/1 -> MATLAB Function2/4(denmEnable)
  Enable_CAM/1 -> MATLAB Function2/3(camEnable)
  Add/1 -> MATLAB Function/1(p), Unit Delay/1
  Demux/1 -> Data/1
  Demux/2 -> Byte/1
  Constant9/1 -> Add/1
  Unit Delay/1 -> Add/2
  denm/1 -> MATLAB Function2/2(denm)
  MATLAB Function/1(z) -> MATLAB Function2/5(z)
  MATLAB Function2/1(outvector_v2x) -> Demux/1
  cam/1 -> MATLAB Function2/1(cam)

== system ASM_Traffic_V2X_Complete_Model_2/IO/V2X_Subsystem/CAM-DENM_Message_Generation/Send_UDP ==
  In1 : Inport
  Input : Inport  Port=2
  Trigger : TriggerPort  VariantControl=Variant  PortDimensions=1
  Display : Display
  Display1 : Display
  UDP Transmit (1)_In : dsmpblib/Data Inport  Priority=10000
      settings: SourceProductName=dSPACE Model Interface Blockset
  UDP Transmit (1)_Out : dsmpblib/Data Outport  Priority=-10000
      settings: SourceProductName=dSPACE Model Interface Blockset
  wires:
  UDP Transmit (1)_In/1 -> Display/1
  UDP Transmit (1)_In/2 -> Display1/1
  In1/1 -> UDP Transmit (1)_Out/1
  Input/1 -> UDP Transmit (1)_Out/2

== system ASM_Traffic_V2X_Complete_Model_2/IO/V2X_Subsystem/Car_Data/EGOCAR_Position ==
  In1 : Inport
  Bus Creator : BusCreator  Inputs=4
  Bus Selector : BusSelector  OutputSignals=Environment.Road.Road_Init.Pos_Vehicle_Init_CoorSys_E[x;y;z][m].Const_Pos_x_Vehicle_Init[m],Environment.Road.Road_Init.Pos_Vehicle_Init_CoorSys_E[x;y;z][m].Const_Pos_y_Vehicle_Init[m],VehicleDynamics.VehicleMovement.Positions.Vehicle.Linear.Pos_Vehicle_CoorSys_E[x;y;z][m].Pos_x_Vehicle_CoorSys_E[m],VehicleDynamics.VehicleMovement.Positions.Vehicle.Linear.Pos_Vehicle_CoorSys_E[x;y;z][m].Pos_y_Vehicle_CoorSys_E[m],VehicleDynamics.VehicleMovement.Positions.Vehicle.Linear.Pos_Vehicle_CoorSys_E[x;y;z][m].Pos_z_Vehicle_CoorSys_E[m],Environment.Road.Pos_Vehicle_GPS[Long;Lat][deg].Longitude[deg],Environment.Road.Pos_Vehicle_GPS[Long;Lat][deg].Latitude[deg]
  Display{,1..4} (5 alike) : Display
  Ego_Lat : Display
  Ego_Long : Display
  Output : Outport
  wires:
  Bus Creator/1 -> Output/1
  Bus Selector/7 -> Ego_Lat/1, Bus Creator/2  "<Latitude[deg]>"
  Bus Selector/4 -> Display3/1, Bus Creator/4  "<Pos_y_Vehicle_CoorSys_E[m]>"
  Bus Selector/5 -> Display4/1  "<Pos_z_Vehicle_CoorSys_E[m]>"
  Bus Selector/6 -> Ego_Long/1, Bus Creator/1  "<Longitude[deg]>"
  Bus Selector/3 -> Display2/1, Bus Creator/3  "<Pos_x_Vehicle_CoorSys_E[m]>"
  Bus Selector/2 -> Display1/1  "<Const_Pos_y_Vehicle_Init[m]>"
  Bus Selector/1 -> Display/1  "<Const_Pos_x_Vehicle_Init[m]>"
  In1/1 -> Bus Selector/1

== system ASM_Traffic_V2X_Complete_Model_2/IO/V2X_Subsystem/Car_Data/Fellow_ID_1 ==
  "EGO_Car_Position " : Inport
  Input : Inport  Port=2
  Bus Creator : BusCreator  Inputs=6
  Bus Creator1 : BusCreator  Inputs=2
  Bus Selector1 : BusSelector  OutputSignals=Environment.Traffic.FellowMovement.FellowPositions.Pos_Fellows_MainPnt_CoorSys_E[x;y;z][m].Pos_x_Fellows[m],Environment.Traffic.FellowMovement.FellowPositions.Pos_Fellows_MainPnt_CoorSys_E[x;y;z][m].Pos_y_Fellows[m],Environment.Traffic.FellowMovement.FellowPositions.Pos_Fellows_MainPnt_CoorSys_E[x;y;z][m].Pos_z_Fellows[m],Environment.Traffic.FellowMovement.FellowVelocities.v_Fellows[x;y;z][km|h],Environment.Traffic.FellowMovement.FellowPositions.Angle_Fellows[x;y;z][deg].Angle_Yaw_Fellows[deg],Environment.Road.UserSignals_Customized.Const_Offset_Lat[deg],Environment.Road.UserSignals_Customized.Const_Offset_Long[deg]
  Display : Display
  Display1 : Display
  Distance_Calculation : Subsystem
  Fellow_ID : Constant
  Fellow_ID_1_Spherical_XY2GPS : Subsystem  TreatAsAtomicUnit=on
  Heading Function : MATLAB Function  TreatAsAtomicUnit=on
  Terminator2 : Terminator
  Variable Selector{,1..3} (4 alike) : dspindex/Variable Selector  NumInputs=1  rowsOrCols=Rows  IdxMode=Variable  Elements=[1 3]  ZerOneIdxMode=One-based  errmode=Clip Index  FillMode=on  FillValues=0
  Output : Outport
  wires:
  Variable Selector3/1 -> Heading Function/1(u)  "Speed"
  Heading Function/1(y) -> Bus Creator/6  "Heading"
  Bus Selector1/5 -> Variable Selector3/1  "<Angle_Yaw_Fellows[deg]>"
  Variable Selector2/1 -> Bus Creator/5  "Speed"
  Bus Selector1/4 -> Variable Selector2/1  "<v_Fellows[x;y;z][km|h]>"
  Bus Selector1/1 -> Variable Selector/1  "<Pos_x_Fellows[m]>"
  Bus Selector1/3 -> Terminator2/1  "<Pos_z_Fellows[m]>"
  Bus Selector1/2 -> Variable Selector1/1  "<Pos_y_Fellows[m]>"
  Input/1 -> Bus Selector1/1
  Distance_Calculation/1(Distance<50m) -> Bus Creator/4  "Enable"
  "EGO_Car_Position "/1 -> Distance_Calculation/3(Egocar)
  Fellow_ID_1_Spherical_XY2GPS/2(Latitude_Veh) -> Bus Creator/2  "Latitude[deg]"
  Fellow_ID/1 -> Variable Selector/2, Variable Selector1/2, Variable Selector2/2, Variable Selector3/2, Bus Creator/3  "Fellow_ID"
  Variable Selector1/1 -> Display1/1, Distance_Calculation/1(Fellow_y), Fellow_ID_1_Spherical_XY2GPS/2(Position_y_Veh)
  Fellow_ID_1_Spherical_XY2GPS/1(Longitude_Veh) -> Bus Creator/1  "Longitude[deg]"
  Bus Creator/1 -> Output/1
  Variable Selector/1 -> Display/1, Distance_Calculation/2(Fellow_x), Fellow_ID_1_Spherical_XY2GPS/1(Position_x_Veh)
  Bus Selector1/6 -> Bus Creator1/1  "<Const_Offset_Lat[deg]>"
  Bus Selector1/7 -> Bus Creator1/2  "<Const_Offset_Long[deg]>"
  Bus Creator1/1 -> Fellow_ID_1_Spherical_XY2GPS/3(Lat_Long)

== system ASM_Traffic_V2X_Complete_Model_2/IO/V2X_Subsystem/Car_Data/Fellow_ID_2 ==
  "EGO_Car_Position " : Inport
  Input : Inport  Port=2
  Bus Creator : BusCreator  Inputs=6
  Bus Creator1 : BusCreator  Inputs=2
  Bus Selector1 : BusSelector  OutputSignals=Environment.Traffic.FellowMovement.FellowPositions.Pos_Fellows_MainPnt_CoorSys_E[x;y;z][m].Pos_x_Fellows[m],Environment.Traffic.FellowMovement.FellowPositions.Pos_Fellows_MainPnt_CoorSys_E[x;y;z][m].Pos_y_Fellows[m],Environment.Traffic.FellowMovement.FellowPositions.Pos_Fellows_MainPnt_CoorSys_E[x;y;z][m].Pos_z_Fellows[m],Environment.Traffic.FellowMovement.FellowVelocities.v_Fellows[x;y;z][km|h],Environment.Traffic.FellowMovement.FellowPositions.Angle_Fellows[x;y;z][deg].Angle_Yaw_Fellows[deg],Environment.Road.UserSignals_Customized.Const_Offset_Lat[deg],Environment.Road.UserSignals_Customized.Const_Offset_Long[deg]
  Display : Display
  Display1 : Display
  Distance_Calculation : Subsystem
  Fellow_ID : Constant  Value=2
  Fellow_ID_1_Spherical_XY2GPS : Subsystem  TreatAsAtomicUnit=on
  Heading Function : MATLAB Function  TreatAsAtomicUnit=on
  Terminator2 : Terminator
  Variable Selector{,1..3} (4 alike) : dspindex/Variable Selector  NumInputs=1  rowsOrCols=Rows  IdxMode=Variable  Elements=[1 3]  ZerOneIdxMode=One-based  errmode=Clip Index  FillMode=on  FillValues=0
  Output : Outport
  wires:
  Variable Selector3/1 -> Heading Function/1(u)  "Speed"
  Heading Function/1(y) -> Bus Creator/6  "Heading"
  Bus Selector1/5 -> Variable Selector3/1  "<Angle_Yaw_Fellows[deg]>"
  Variable Selector2/1 -> Bus Creator/5  "Speed"
  Bus Selector1/4 -> Variable Selector2/1  "<v_Fellows[x;y;z][km|h]>"
  Bus Selector1/1 -> Variable Selector/1  "<Pos_x_Fellows[m]>"
  Bus Selector1/3 -> Terminator2/1  "<Pos_z_Fellows[m]>"
  Bus Selector1/2 -> Variable Selector1/1  "<Pos_y_Fellows[m]>"
  Input/1 -> Bus Selector1/1
  Distance_Calculation/1(Distance<50m) -> Bus Creator/4  "Enable"
  "EGO_Car_Position "/1 -> Distance_Calculation/3(Egocar)
  Fellow_ID_1_Spherical_XY2GPS/2(Latitude_Veh) -> Bus Creator/2  "Latitude[deg]"
  Fellow_ID/1 -> Variable Selector/2, Variable Selector1/2, Variable Selector2/2, Variable Selector3/2, Bus Creator/3  "Fellow_ID"
  Variable Selector1/1 -> Display1/1, Distance_Calculation/1(Fellow_y), Fellow_ID_1_Spherical_XY2GPS/2(Position_y_Veh)
  Fellow_ID_1_Spherical_XY2GPS/1(Longitude_Veh) -> Bus Creator/1  "Longitude[deg]"
  Bus Creator/1 -> Output/1
  Variable Selector/1 -> Display/1, Distance_Calculation/2(Fellow_x), Fellow_ID_1_Spherical_XY2GPS/1(Position_x_Veh)
  Bus Selector1/6 -> Bus Creator1/1  "<Const_Offset_Lat[deg]>"
  Bus Selector1/7 -> Bus Creator1/2  "<Const_Offset_Long[deg]>"
  Bus Creator1/1 -> Fellow_ID_1_Spherical_XY2GPS/3(Lat_Long)
